simulink model "DSP_PROJECT"  (R2025a)
settings: Solver=ode4  StartTime=0.0  StopTime=50  FixedStep=0.001  RelTol=1e-3
values from neighbouring files (symbols this model uses):
  a_fir = 1    [DSP_PROJECT_FIR.m]
  b_fir = fir1(fir_order, Wn_fir, 'low', hamming(fir_order+1))    [DSP_PROJECT_FIR.m]
undefined symbols (not defined in the file or in its folder): a, b, dspblkCoreblockFVToolHelper, gcbh
libraries: eeGeneralControl x1
settings Model: Creator=user  LastModifiedBy=Usuario
settings DebuggingCC: UnconnectedInputMsg=warning  UnconnectedOutputMsg=warning  UnconnectedLineMsg=warning
settings ModelReferenceCC: EnableRefExpFcnMdlSchedulingChecks=on
settings RTWCC: GPUComputeCapability=3.5  DLArmComputeVersion=19.05

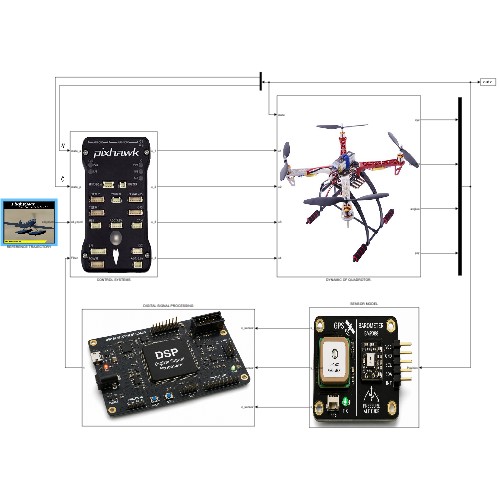
[thumbnail: Simulink's stored preview of the top-level diagram]
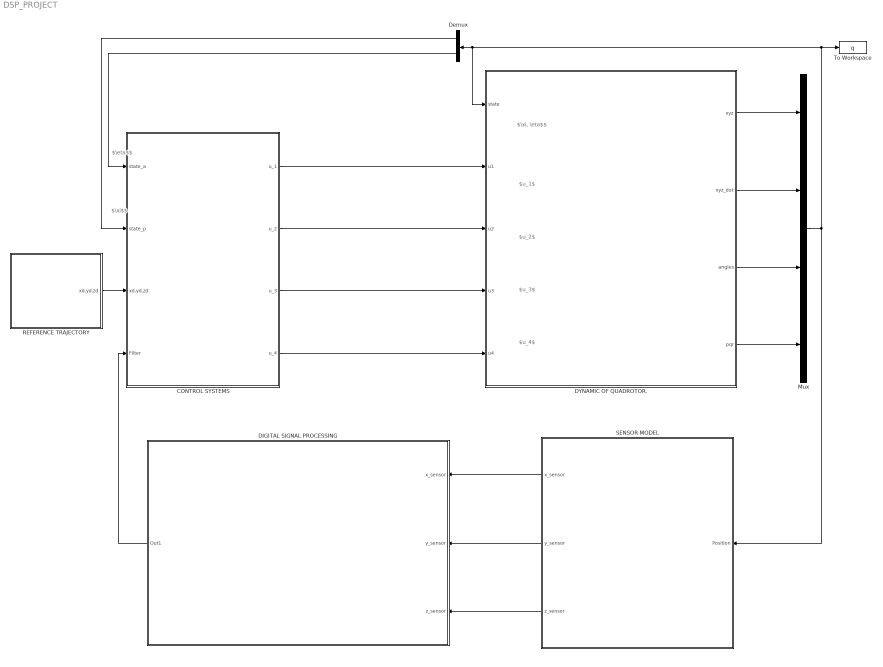
== system DSP_PROJECT ==
  note: $u_1$
  note: $\xi$$
  note: $\eta$$
  note: $\xi, \eta$$
  note: $u_2$
  note: $u_3$
  note: $u_4$
  CONTROL SYSTEMS : Subsystem
      mask Display: image('pixhawk.png');
  DIGITAL SIGNAL PROCESSING : Subsystem
      mask Display: image('DSP.png');
  DYNAMIC OF QUADROTOR. : Subsystem
      mask Display: image('droneHardware.jpeg');
  Demux : Demux  Outputs=[6 6]
  Mux : Mux
  REFERENCE TRAJECTORY : Subsystem
      mask Display: image('FlightGear.png');
  SENSOR MODEL : Subsystem
      mask Display: image('SENSOR.png');
  To Workspace : ToWorkspace  VariableName=q  SampleTime=-1
  wires:
  Demux/1 -> CONTROL SYSTEMS/2(state_p)
  Demux/2 -> CONTROL SYSTEMS/1(state_a)
  CONTROL SYSTEMS/1(u_1) -> DYNAMIC OF QUADROTOR./2(u1)
  CONTROL SYSTEMS/2(u_2) -> DYNAMIC OF QUADROTOR./3(u2)
  CONTROL SYSTEMS/3(u_3) -> DYNAMIC OF QUADROTOR./4(u3)
  CONTROL SYSTEMS/4(u_4) -> DYNAMIC OF QUADROTOR./5(u4)
  REFERENCE TRAJECTORY/1(xd,yd,zd) -> CONTROL SYSTEMS/3(xd,yd,zd)
  DYNAMIC OF QUADROTOR./1(xyz) -> Mux/1
  DYNAMIC OF QUADROTOR./2(xyz_dot) -> Mux/2
  DYNAMIC OF QUADROTOR./3(angles) -> Mux/3
  DYNAMIC OF QUADROTOR./4(pqr) -> Mux/4
  Mux/1 -> SENSOR MODEL/1(Position), DYNAMIC OF QUADROTOR./1(state), Demux/1, To Workspace/1
  SENSOR MODEL/1(x_sensor) -> DIGITAL SIGNAL PROCESSING/1(x_sensor)
  SENSOR MODEL/2(y_sensor) -> DIGITAL SIGNAL PROCESSING/2(y_sensor)
  SENSOR MODEL/3(z_sensor) -> DIGITAL SIGNAL PROCESSING/3(z_sensor)
  DIGITAL SIGNAL PROCESSING/1(Out1) -> CONTROL SYSTEMS/4(Filter)

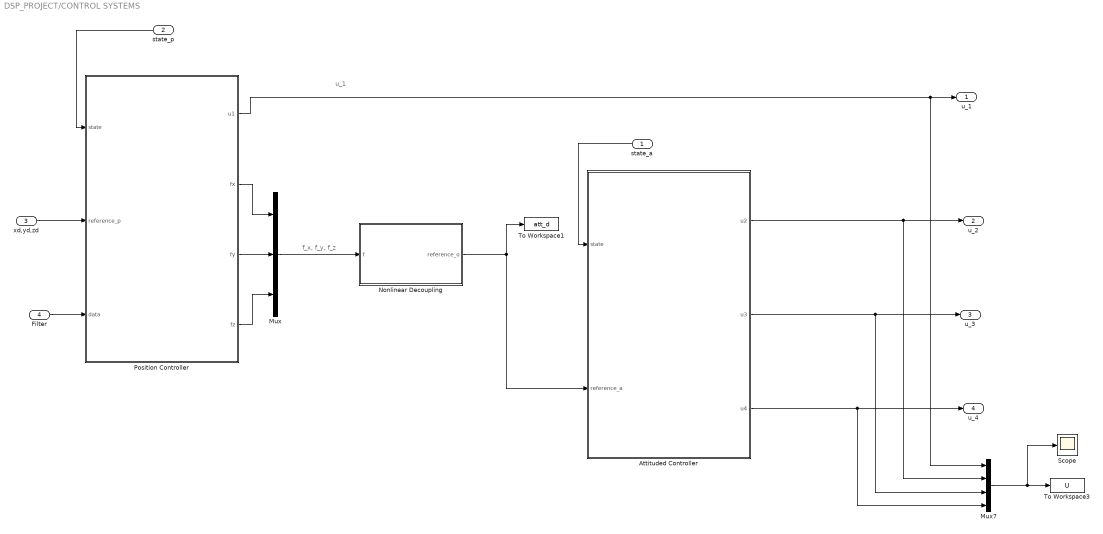
== system DSP_PROJECT/CONTROL SYSTEMS ==
  note: f_x, f_y, f_z
  note: u_1
  state_a : Inport
  state_p : Inport  Port=2
  xd,yd,zd : Inport  Port=3
  Filter : Inport  Port=4
  Attituded Controller : MATLAB Function  TreatAsAtomicUnit=on
  Mux : Mux  Inputs=3
  Mux7 : Mux
  Nonlinear Decoupling : MATLAB Function  TreatAsAtomicUnit=on
  Position Controller : MATLAB Function  TreatAsAtomicUnit=on
  Scope : Scope
      settings: ActiveDisplayYMinimum=-1  ActiveDisplayYMaximum=1
  To Workspace1 : ToWorkspace  VariableName=att_d  SampleTime=-1
  To Workspace3 : ToWorkspace  VariableName=U  SampleTime=-1
  u_1 : Outport
  u_2 : Outport  Port=2
  u_3 : Outport  Port=3
  u_4 : Outport  Port=4
  wires:
  Mux7/1 -> Scope/1, To Workspace3/1
  state_a/1 -> Attituded Controller/1(state)
  Nonlinear Decoupling/1(reference_o) -> To Workspace1/1, Attituded Controller/2(reference_a)
  Attituded Controller/3(u4) -> u_4/1, Mux7/4
  Attituded Controller/2(u3) -> u_3/1, Mux7/3
  Attituded Controller/1(u2) -> u_2/1, Mux7/2
  Position Controller/1(u1) -> Mux7/1, u_1/1
  state_p/1 -> Position Controller/1(state)
  xd,yd,zd/1 -> Position Controller/2(reference_p)
  Position Controller/2(fx) -> Mux/1
  Position Controller/3(fy) -> Mux/2
  Position Controller/4(fz) -> Mux/3
  Mux/1 -> Nonlinear Decoupling/1(f)
  Filter/1 -> Position Controller/3(data)

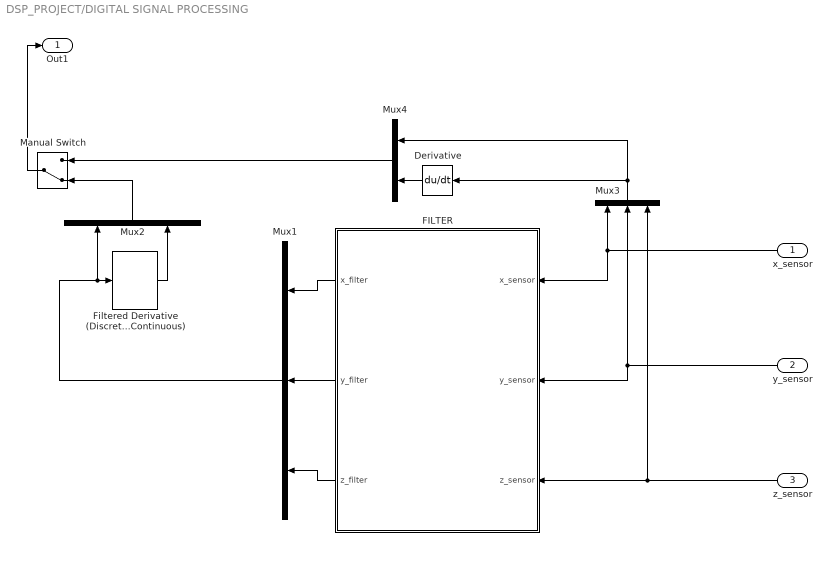
== system DSP_PROJECT/DIGITAL SIGNAL PROCESSING ==
  x_sensor : Inport
  y_sensor : Inport  Port=2
  z_sensor : Inport  Port=3
  Derivative : Derivative
  FILTER : Subsystem
  Filtered Derivative (Discrete or Continuous) : eeGeneralControl/Filtered Derivative (Discrete or Continuous)  K=1  T=0.1  B=inf  A=-inf  minRatio=10  init_option=Inherited from block input  x0=0  Ts=0.001
      settings: LibrarySourceBlock=|
      | ee_sl_lib/General Control/Filtered Derivative
      | (Discrete or Continuous)
  Manual Switch : ManualSwitch  CurrentSetting=0
  Mux1 : Mux  Inputs=3
  Mux2 : Mux  Inputs=2
  Mux3 : Mux  Inputs=3
  Mux4 : Mux  Inputs=2
  Out1 : Outport
  wires:
  FILTER/3(z_filter) -> Mux1/3
  Mux1/1 -> Filtered Derivative (Discrete or Continuous)/1, Mux2/1
  Filtered Derivative (Discrete or Continuous)/1 -> Mux2/2
  y_sensor/1 -> FILTER/2(y_sensor), Mux3/2
  z_sensor/1 -> FILTER/3(z_sensor), Mux3/3
  FILTER/2(y_filter) -> Mux1/2
  x_sensor/1 -> FILTER/1(x_sensor), Mux3/1
  Mux3/1 -> Mux4/1, Derivative/1
  FILTER/1(x_filter) -> Mux1/1
  Mux2/1 -> Manual Switch/2
  Derivative/1 -> Mux4/2
  Mux4/1 -> Manual Switch/1
  Manual Switch/1 -> Out1/1

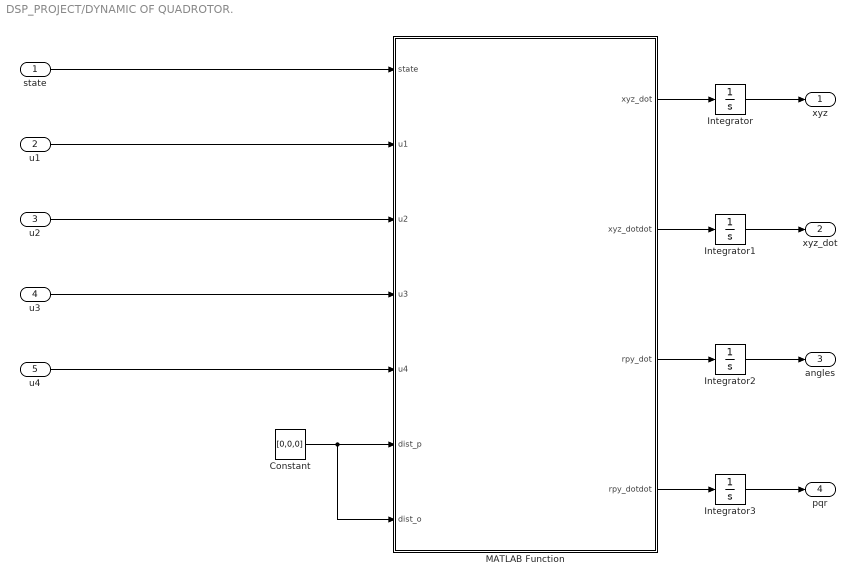
== system DSP_PROJECT/DYNAMIC OF QUADROTOR. ==
  state : Inport
  u1 : Inport  Port=2
  u2 : Inport  Port=3
  u3 : Inport  Port=4
  u4 : Inport  Port=5
  Constant : Constant  Value=[0,0,0]
  Integrator : Integrator  InitialCondition=[1 1 0.01]
  Integrator1 : Integrator  InitialCondition=[0.01 0.01 0.01]
  Integrator2 : Integrator  InitialCondition=[0.01 0.01 0.01]
  Integrator3 : Integrator  InitialCondition=[0.01 0.01 0.01]
  MATLAB Function : MATLAB Function  TreatAsAtomicUnit=on
  xyz : Outport
  xyz_dot : Outport  Port=2
  angles : Outport  Port=3
  pqr : Outport  Port=4
  wires:
  MATLAB Function/1(xyz_dot) -> Integrator/1
  Integrator/1 -> xyz/1
  state/1 -> MATLAB Function/1(state)
  u1/1 -> MATLAB Function/2(u1)
  u2/1 -> MATLAB Function/3(u2)
  u3/1 -> MATLAB Function/4(u3)
  u4/1 -> MATLAB Function/5(u4)
  Constant/1 -> MATLAB Function/7(dist_o), MATLAB Function/6(dist_p)
  MATLAB Function/2(xyz_dotdot) -> Integrator1/1
  Integrator1/1 -> xyz_dot/1
  Integrator2/1 -> angles/1
  MATLAB Function/3(rpy_dot) -> Integrator2/1
  Integrator3/1 -> pqr/1
  MATLAB Function/4(rpy_dotdot) -> Integrator3/1

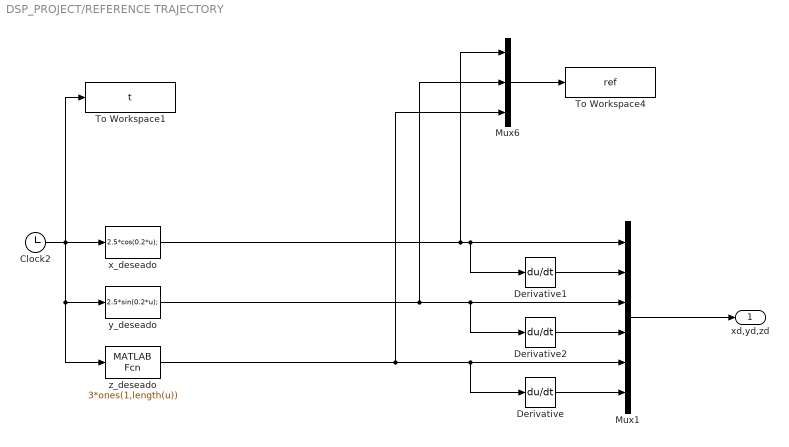
== system DSP_PROJECT/REFERENCE TRAJECTORY ==
  Clock2 : Clock
  Derivative : Derivative
  Derivative1 : Derivative
  Derivative2 : Derivative
  Mux1 : Mux  Inputs=6
  Mux6 : Mux  Inputs=3
  To Workspace1 : ToWorkspace  VariableName=t  SampleTime=-1
  To Workspace4 : ToWorkspace  VariableName=ref  SampleTime=-1
  x_deseado : MATLABFcn  MATLABFcn=2.5*cos(0.2*u);
  y_deseado : MATLABFcn  MATLABFcn=2.5*sin(0.2*u);
  z_deseado : MATLABFcn  MATLABFcn=3*ones(1,length(u))
  xd,yd,zd : Outport
  wires:
  Mux6/1 -> To Workspace4/1
  z_deseado/1 -> Derivative/1, Mux1/5, Mux6/3
  Derivative1/1 -> Mux1/2
  y_deseado/1 -> Derivative2/1, Mux1/3, Mux6/2
  Clock2/1 -> x_deseado/1, z_deseado/1, y_deseado/1, To Workspace1/1
  Derivative2/1 -> Mux1/4
  Derivative/1 -> Mux1/6
  x_deseado/1 -> Mux1/1, Derivative1/1, Mux6/1
  Mux1/1 -> xd,yd,zd/1

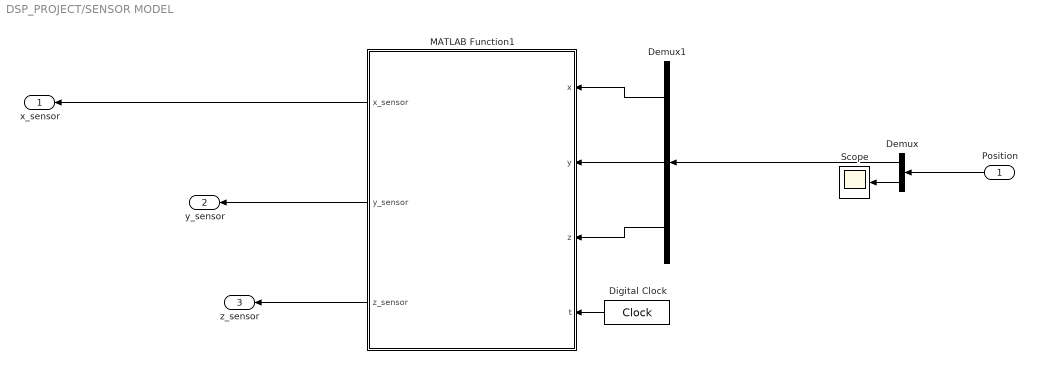
== system DSP_PROJECT/SENSOR MODEL ==
  Position : Inport
  Demux : Demux  Outputs=[3 9]
  Demux1 : Demux  Outputs=3
  Digital Clock : DigitalClock  SampleTime=0.001
  MATLAB Function1 : MATLAB Function  TreatAsAtomicUnit=on
  Scope : Scope
  x_sensor : Outport
  y_sensor : Outport  Port=2
  z_sensor : Outport  Port=3
  wires:
  MATLAB Function1/1(x_sensor) -> x_sensor/1
  Demux1/3 -> MATLAB Function1/3(z)
  Demux1/2 -> MATLAB Function1/2(y)
  Digital Clock/1 -> MATLAB Function1/4(t)
  Demux1/1 -> MATLAB Function1/1(x)
  MATLAB Function1/2(y_sensor) -> y_sensor/1
  MATLAB Function1/3(z_sensor) -> z_sensor/1
  Position/1 -> Demux/1
  Demux/1 -> Demux1/1
  Demux/2 -> Scope/1

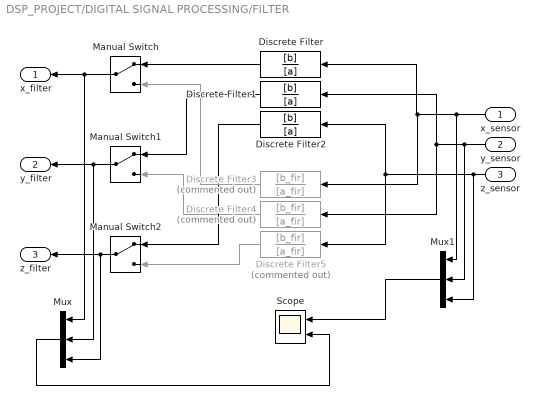
== system DSP_PROJECT/DIGITAL SIGNAL PROCESSING/FILTER ==
  x_sensor : Inport
  y_sensor : Inport  Port=2
  z_sensor : Inport  Port=3
  Discrete Filter : DiscreteFilter  LoadFcn=dspblkCoreblockFVToolHelper(gcbh,'load');  Numerator=[b]  Denominator=[a]
      settings: CopyFcn=dspblkCoreblockFVToolHelper(gcbh,'copy');  DeleteFcn=dspblkCoreblockFVToolHelper(gcbh,'close');  ModelCloseFcn=dspblkCoreblockFVToolHelper(gcbh,'close');  PreSaveFcn=dspblkCoreblockFVToolHelper(gcbh,'presave');  PostSaveFcn=dspblkCoreblockFVToolHelper(gcbh,'postsave');  CloseFcn=dspblkCoreblockFVToolHelper(gcbh,'close');
  Discrete Filter1 : DiscreteFilter  LoadFcn=dspblkCoreblockFVToolHelper(gcbh,'load');  Numerator=[b]  Denominator=[a]
      settings: CopyFcn=dspblkCoreblockFVToolHelper(gcbh,'copy');  DeleteFcn=dspblkCoreblockFVToolHelper(gcbh,'close');  ModelCloseFcn=dspblkCoreblockFVToolHelper(gcbh,'close');  PreSaveFcn=dspblkCoreblockFVToolHelper(gcbh,'presave');  PostSaveFcn=dspblkCoreblockFVToolHelper(gcbh,'postsave');  CloseFcn=dspblkCoreblockFVToolHelper(gcbh,'close');
  Discrete Filter2 : DiscreteFilter  LoadFcn=dspblkCoreblockFVToolHelper(gcbh,'load');  Numerator=[b]  Denominator=[a]
      settings: CopyFcn=dspblkCoreblockFVToolHelper(gcbh,'copy');  DeleteFcn=dspblkCoreblockFVToolHelper(gcbh,'close');  ModelCloseFcn=dspblkCoreblockFVToolHelper(gcbh,'close');  PreSaveFcn=dspblkCoreblockFVToolHelper(gcbh,'presave');  PostSaveFcn=dspblkCoreblockFVToolHelper(gcbh,'postsave');  CloseFcn=dspblkCoreblockFVToolHelper(gcbh,'close');
  Discrete Filter3 : DiscreteFilter  Commented=on  LoadFcn=dspblkCoreblockFVToolHelper(gcbh,'load');  Numerator=[b_fir]  Denominator=[a_fir]
      settings: CopyFcn=dspblkCoreblockFVToolHelper(gcbh,'copy');  DeleteFcn=dspblkCoreblockFVToolHelper(gcbh,'close');  ModelCloseFcn=dspblkCoreblockFVToolHelper(gcbh,'close');  PreSaveFcn=dspblkCoreblockFVToolHelper(gcbh,'presave');  PostSaveFcn=dspblkCoreblockFVToolHelper(gcbh,'postsave');  CloseFcn=dspblkCoreblockFVToolHelper(gcbh,'close');
  Discrete Filter4 : DiscreteFilter  Commented=on  LoadFcn=dspblkCoreblockFVToolHelper(gcbh,'load');  Numerator=[b_fir]  Denominator=[a_fir]
      settings: CopyFcn=dspblkCoreblockFVToolHelper(gcbh,'copy');  DeleteFcn=dspblkCoreblockFVToolHelper(gcbh,'close');  ModelCloseFcn=dspblkCoreblockFVToolHelper(gcbh,'close');  PreSaveFcn=dspblkCoreblockFVToolHelper(gcbh,'presave');  PostSaveFcn=dspblkCoreblockFVToolHelper(gcbh,'postsave');  CloseFcn=dspblkCoreblockFVToolHelper(gcbh,'close');
  Discrete Filter5 : DiscreteFilter  Commented=on  LoadFcn=dspblkCoreblockFVToolHelper(gcbh,'load');  Numerator=[b_fir]  Denominator=[a_fir]
      settings: CopyFcn=dspblkCoreblockFVToolHelper(gcbh,'copy');  DeleteFcn=dspblkCoreblockFVToolHelper(gcbh,'close');  ModelCloseFcn=dspblkCoreblockFVToolHelper(gcbh,'close');  PreSaveFcn=dspblkCoreblockFVToolHelper(gcbh,'presave');  PostSaveFcn=dspblkCoreblockFVToolHelper(gcbh,'postsave');  CloseFcn=dspblkCoreblockFVToolHelper(gcbh,'close');
  Manual Switch : ManualSwitch
  Manual Switch1 : ManualSwitch
  Manual Switch2 : ManualSwitch
  Mux : Mux  Inputs=3
  Mux1 : Mux  Inputs=3
  Scope : Scope  NumInputPorts=2
      settings: ActiveDisplayYMinimum=-3.5527443324160544  ActiveDisplayYMaximum=3.8628754450907112  DataLoggingVariableName=ScopeData3
  x_filter : Outport
  y_filter : Outport  Port=2
  z_filter : Outport  Port=3
  wires:
  x_sensor/1 -> Mux1/1, Discrete Filter3/1, Discrete Filter/1
  Discrete Filter1/1 -> Manual Switch1/1
  Discrete Filter4/1 -> Manual Switch1/2
  Discrete Filter2/1 -> Manual Switch2/1
  Manual Switch1/1 -> Mux/2, y_filter/1
  y_sensor/1 -> Mux1/2, Discrete Filter4/1, Discrete Filter1/1
  Manual Switch2/1 -> Mux/3, z_filter/1
  z_sensor/1 -> Mux1/3, Discrete Filter5/1, Discrete Filter2/1
  Discrete Filter/1 -> Manual Switch/1
  Discrete Filter3/1 -> Manual Switch/2
  Discrete Filter5/1 -> Manual Switch2/2
  Manual Switch/1 -> Mux/1, x_filter/1
  Mux1/1 -> Scope/1
  Mux/1 -> Scope/2

== matlab function DSP_PROJECT/CONTROL SYSTEMS/Position Controller ==
  data: state input; u1 output; reference_p input; fx output; fy output; fz output; data input
function [u1,fx,fy,fz] = Position_Control(state,reference_p, data)
%% Parametros Quadrotor
    m=1.636;
    g=9.8;
    Jx=0.0232;
    Jy=0.0249;
    Jz=0.0342;  
%% Estados
x = data(1); x_dot = data(4);
y = data(2); y_dot = data(5);
z = data(3); z_dot = data(6);

% x = state(1); x_dot = state(4);
% y = state(2); y_dot = state(5);
% z = state(3); z_dot = state(6);

%% Posiciones deseadas
    xd=reference_p(1); %x
    xd_dot=reference_p(2);
    xd_dotdot=0;
    yd=reference_p(3);  %y
    yd_dot=reference_p(4);
    yd_dotdot=0;
    zd=reference_p(5);  %z
    zd_dot=reference_p(6);
    zd_dotdot=0;

%% POSITION
    %% Parameters
c=1.2;
mu1=0;
mu2=5.5*0.1;
   %% ERRORES POSICION
    e1x=x-xd;
    e1y=y-yd;
    e1z=z-zd;
    e1x_dot=x_dot-xd_dot;
    e1y_dot=y_dot-yd_dot;
    e1z_dot=z_dot-zd_dot;
    %% design
    sx=e1x_dot + c*e1x ;
    sy=e1y_dot + c*e1y ;
    sz=e1z_dot + c*e1z ;
    %% Adaptive
    fx=(xd_dotdot - c*e1x_dot - mu1*sx - mu2*tanh(sx));
    fy=(yd_dotdot - c*e1y_dot - mu1*sy - mu2*tanh(sy));
    fz=(zd_dotdot - c*e1z_dot - mu1*sz - mu2*tanh(sz));
 
    u1=m*sqrt(fx.^2+fy.^2+(fz+g).^2);
end

== matlab function DSP_PROJECT/DYNAMIC OF QUADROTOR./MATLAB Function ==
  data: state input; xyz_dot output; u1 input; u2 input; u3 input; u4 input; dist_p input; dist_o input; xyz_dotdot output; rpy_dot output; rpy_dotdot output
function [xyz_dot,xyz_dotdot,rpy_dot,rpy_dotdot] = Dynamic_Quadrotor(state,u1,u2,u3,u4,dist_p, dist_o)
%% Parametros del Quadrotor UAV
    mq=1.636;
    g=9.8;
    Jx=0.0232;
    Jy=0.0249;
    Jz=0.0342;

%% Estados
x = state(1); x_dot = state(4);
y = state(2); y_dot = state(5);
z = state(3); z_dot = state(6);

phi = state(7);   phi_dot = state(10);
theta = state(8); theta_dot = state(11);
psi = state(9);   psi_dot = state(12);

%% Entradas
Uq1=[u1,u2,u3,u4];
dx=dist_p(1); dy=dist_p(2);  dz=dist_p(3);
dphi=dist_o(1); dtheta=dist_o(2);  dpsi=dist_o(3);

%% Aceleraciones
x_dotdot=(cos(phi)*sin(theta)*cos(psi)+sin(phi)*sin(psi))*(Uq1(1)/mq) ;
y_dotdot=(cos(phi)*sin(theta)*sin(psi)-sin(phi)*cos(psi))*(Uq1(1)/mq) ;
z_dotdot=(cos(phi)*cos(theta))*Uq1(1)/mq -g ;
phi_dotdot=((Jy-Jz)/Jx)*theta_dot*psi_dot+Uq1(2)/Jx;
theta_dotdot=((Jz-Jx)/Jy)*phi_dot*psi_dot+Uq1(3)/Jy;
psi_dotdot=((Jx-Jy)/Jz)*theta_dot*phi_dot+Uq1(4)/Jz;

%%
xyz_dotdot=[x_dotdot;y_dotdot;z_dotdot];
rpy_dotdot=[phi_dotdot;theta_dotdot;psi_dotdot];
xyz_dot=[x_dot;y_dot;z_dot];
rpy_dot=[phi_dot;theta_dot;psi_dot];

end

== matlab function DSP_PROJECT/CONTROL SYSTEMS/Attituded Controller ==
  data: state input; u2 output; reference_a input; u3 output; u4 output
function [u2,u3,u4] = Attituded_Control(state,reference_a)
%% Parametros Quadrotor 1
    g=9.8;
    Jx=0.0232;
    Jy=0.0249;
    Jz=0.0342; 
%% Estados
phi = state(1);   phi_dot = state(4);
theta = state(2); theta_dot = state(5);
psi = state(3);   psi_dot = state(6);

%% Posiciones deseadas
    phid=reference_a(1);   %phi
    phid_dot=0;
    phid_dotdot=0;
    thetad=reference_a(2);   %theta
    thetad_dot=0;
    thetad_dotdot=0;
    psid=0;   %yaw
    psid_dot=0;
    psid_dotdot=0; 
    
    
%% ACTITUD
%% functions
    fphi = theta_dot*psi_dot*(Jy - Jz)/Jx;
    gphi = 1/Jx;
    ftheta = phi_dot*psi_dot*(Jz - Jx)/Jy;
    gtheta = 1/Jy;
    fpsi = phi_dot*theta_dot*(Jx - Jy)/Jz;
    gpsi = 1/Jz;
    
    %% ERRORES ACTITUD
     ephi = (phi - phid);
     ephi_dot = (phi_dot - phid_dot);
     etheta = (theta - thetad);
     etheta_dot = (theta_dot - thetad_dot);
     epsi = (psi - psid);
     epsi_dot = (psi_dot - psid_dot);
      
    %% parameters
    cphi=12;
    ctheta=12;
    cpsi=12;
    c2=0.7;
    c3=10;
    
    %% Design
    sphi=ephi_dot + cphi*ephi;
    stheta=etheta_dot + ctheta*etheta;
    spsi=epsi_dot + cpsi*epsi;
    
    u2=(1/gphi)*(phid_dotdot - fphi - cphi*ephi_dot  - c2*tanh(sphi) - c3*sphi);
    u3=(1/gtheta)*(thetad_dotdot - ftheta - ctheta*etheta_dot  - c2*tanh(stheta) - c3*stheta);
    u4=(1/gpsi)*(psid_dotdot - fpsi - cpsi*epsi_dot  - c2*tanh(spsi) - c3*spsi);
    
end

== matlab function DSP_PROJECT/CONTROL SYSTEMS/Nonlinear Decoupling ==
  data: f input; reference_o output
function reference_o =Decoupling(f)

fx=f(1);
fy=f(2);
fz=f(3);
m=1.636;
g=9.8;
psid=0;
u1=m*sqrt(fx.^2+fy.^2+(fz+g).^2);

    % Phi_d y Theta_d
    phid=asin((m*(fx*sin(psid)-fy*cos(psid)))/(u1));
    thetad=atan((fx*cos(psid)+fy*sin(psid))/(fz+g));
    
reference_o=[phid,thetad];

== matlab function DSP_PROJECT/SENSOR MODEL/MATLAB Function1 ==
  settings: updateMethod=DISCRETE  sampleTime=0.001
  data: x input; x_sensor output; y input; z input; y_sensor output; z_sensor output; t input
function [x_sensor, y_sensor, z_sensor] = sensor_model_quad(x, y, z,t)
%#codegen
% SENSOR_MODEL_QUAD


%% ========================================================
% PARAMETROS DEL SENSOR DE POSICION (GPS / BAROMETRO)
% =========================================================
% 1) SENSOR PARAMETERS

% GPS model for x and y
bias_x = 0.02;      % [m]
bias_y = -0.015;    % [m]
sigma_x = 0.05;     % [m]
sigma_y = 0.05;     % [m]

% Barometer model for z
bias_z = 0.03;      % [m]
sigma_z = 0.03;     % [m]

% High-frequency sinusoidal disturbance
A_x = 0.03;         % [m]
A_y = 0.03;         % [m]
A_z = 0.02;         % [m]

f_x = 20;           % [Hz]
f_y = 25;           % [Hz]
f_z = 15;           % [Hz]


% 2) RANDOM NOISE
nx = sigma_x * randn;
ny = sigma_y * randn;
nz = sigma_z * randn;


% 3) SINUSOIDAL DISTURBANCE
dx = A_x * sin(2*pi*f_x*t);
dy = A_y * sin(2*pi*f_y*t);
dz = A_z * sin(2*pi*f_z*t);

% 4) SENSOR MEASUREMENTS
x_sensor = x + bias_x + nx + dx;
y_sensor = y + bias_y + ny + dy;
z_sensor = z + bias_z + nz + dz;

end
